simulink model "SMC_KI_s"  (R2023a)
settings: Solver=VariableStepAuto  StartTime=0.0  StopTime=10.0  RelTol=1e-3
undefined symbols (not defined in the file): C_col, DiscIntNeverNeededParam, J_col, K, k_I, k_sw, lambda, Phi, Tamax_table, Tamax_v_bp_ms, tau_f, Ts_ctrl
settings Model: Creator=Tan_Tram  LastModifiedBy=Tan_Tram

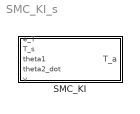
== system SMC_KI_s ==
  SMC_KI : Subsystem

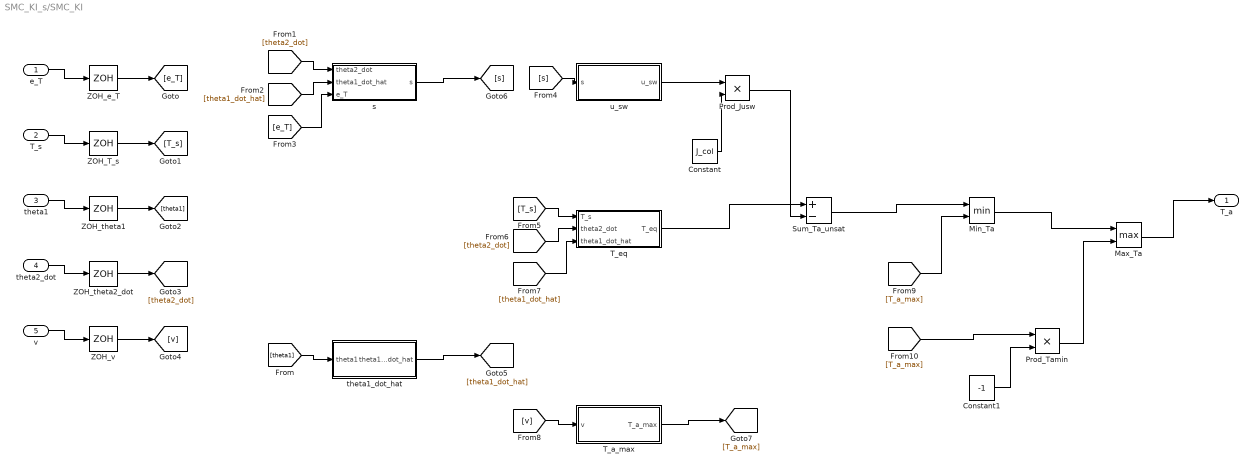
== system SMC_KI_s/SMC_KI ==
  e_T : Inport
  T_s : Inport  Port=2
  theta1 : Inport  Port=3
  theta2_dot : Inport  Port=4
  v : Inport  Port=5
  Constant : Constant  Value=J_col
  Constant1 : Constant  Value=-1
  Max_Ta : MinMax  Function=max  Inputs=2
  Min_Ta : MinMax  Inputs=2
  Prod_Jusw : Product  Inputs=**
  Prod_Tamin : Product  Inputs=**
  Sum_Ta_unsat : Sum  Inputs=+-
  T_a_max : Subsystem
  T_eq : Subsystem
  ZOH_T_s : ZeroOrderHold  SampleTime=Ts_ctrl
  ZOH_e_T : ZeroOrderHold  SampleTime=Ts_ctrl
  ZOH_theta1 : ZeroOrderHold  SampleTime=Ts_ctrl
  ZOH_theta2_dot : ZeroOrderHold  SampleTime=Ts_ctrl
  ZOH_v : ZeroOrderHold  SampleTime=Ts_ctrl
  s : Subsystem
  theta1_dot_hat : Subsystem
  u_sw : Subsystem
  T_a : Outport
  wires:
  e_T/1 -> ZOH_e_T/1
  ZOH_e_T/1 -> [e_T]
  T_s/1 -> ZOH_T_s/1
  ZOH_T_s/1 -> [T_s]
  theta1/1 -> ZOH_theta1/1
  ZOH_theta1/1 -> [theta1]
  theta2_dot/1 -> ZOH_theta2_dot/1
  ZOH_theta2_dot/1 -> [theta2_dot]
  v/1 -> ZOH_v/1
  ZOH_v/1 -> [v]
  [theta1] -> theta1_dot_hat/1(theta1)
  theta1_dot_hat/1(theta1_dot_hat) -> [theta1_dot_hat]
  [theta2_dot] -> s/1(theta2_dot)
  [theta1_dot_hat] -> s/2(theta1_dot_hat)
  [e_T] -> s/3(e_T)
  s/1(s) -> [s]
  [s] -> u_sw/1(s)
  [T_s] -> T_eq/1(T_s)
  [theta2_dot] -> T_eq/2(theta2_dot)
  [theta1_dot_hat] -> T_eq/3(theta1_dot_hat)
  u_sw/1(u_sw) -> Prod_Jusw/1
  Constant/1 -> Prod_Jusw/2
  T_eq/1(T_eq) -> Sum_Ta_unsat/1
  Prod_Jusw/1 -> Sum_Ta_unsat/2
  [v] -> T_a_max/1(v)
  T_a_max/1(T_a_max) -> [T_a_max]
  Sum_Ta_unsat/1 -> Min_Ta/1
  [T_a_max] -> Min_Ta/2
  [T_a_max] -> Prod_Tamin/1
  Constant1/1 -> Prod_Tamin/2
  Min_Ta/1 -> Max_Ta/1
  Prod_Tamin/1 -> Max_Ta/2
  Max_Ta/1 -> T_a/1

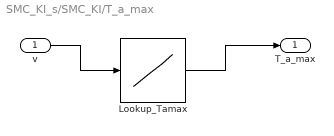
== system SMC_KI_s/SMC_KI/T_a_max ==
  v : Inport
  Lookup_Tamax : Lookup_n-D  NumberOfTableDimensions=1  BreakpointsForDimension1=Tamax_v_bp_ms  BreakpointsForDimension3=[5, 7]  Table=Tamax_table  ExtrapMethod=Clip  InternalRulePriority=Speed  RndMeth=Simplest
  T_a_max : Outport
  wires:
  v/1 -> Lookup_Tamax/1
  Lookup_Tamax/1 -> T_a_max/1

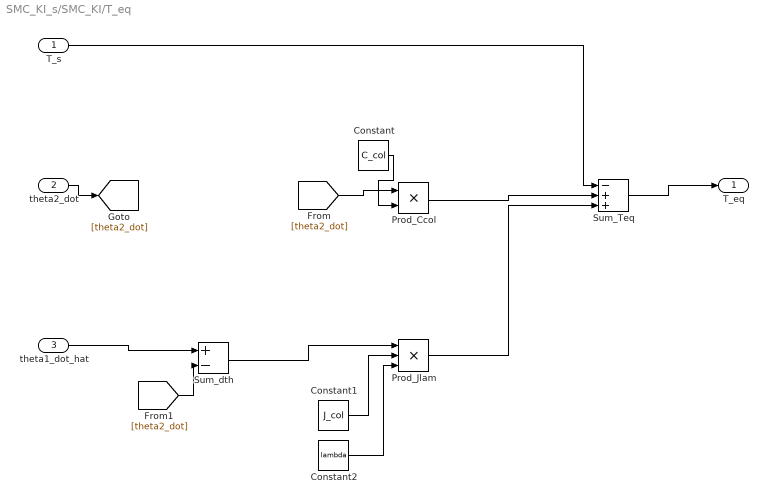
== system SMC_KI_s/SMC_KI/T_eq ==
  T_s : Inport
  theta2_dot : Inport  Port=2
  theta1_dot_hat : Inport  Port=3
  Constant : Constant  Value=C_col
  Constant1 : Constant  Value=J_col
  Constant2 : Constant  Value=lambda
  Prod_Ccol : Product  Inputs=**
  Prod_Jlam : Product  Inputs=***
  Sum_Teq : Sum  Inputs=-++
  Sum_dth : Sum  Inputs=+-
  T_eq : Outport
  wires:
  theta2_dot/1 -> [theta2_dot]
  [theta2_dot] -> Prod_Ccol/1
  Constant/1 -> Prod_Ccol/2
  theta1_dot_hat/1 -> Sum_dth/1
  [theta2_dot] -> Sum_dth/2
  Sum_dth/1 -> Prod_Jlam/1
  Constant1/1 -> Prod_Jlam/2
  Constant2/1 -> Prod_Jlam/3
  T_s/1 -> Sum_Teq/1
  Prod_Ccol/1 -> Sum_Teq/2
  Prod_Jlam/1 -> Sum_Teq/3
  Sum_Teq/1 -> T_eq/1

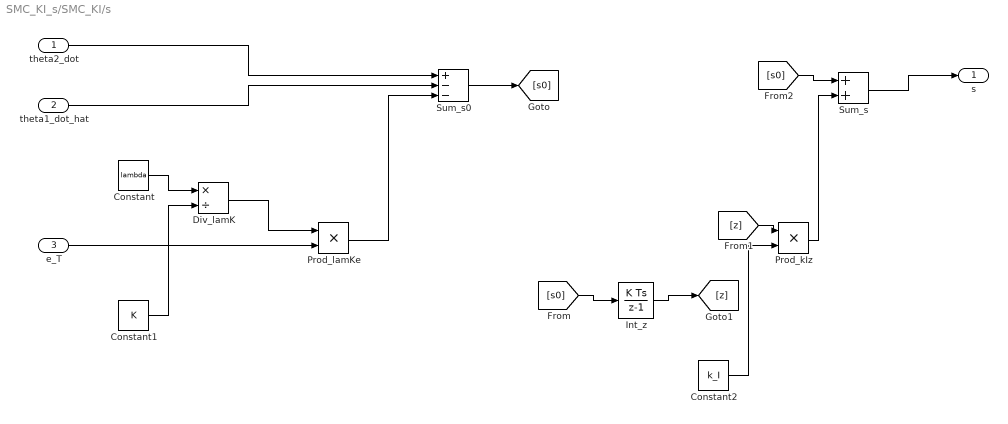
== system SMC_KI_s/SMC_KI/s ==
  theta2_dot : Inport
  theta1_dot_hat : Inport  Port=2
  e_T : Inport  Port=3
  Constant : Constant  Value=lambda
  Constant1 : Constant  Value=K
  Constant2 : Constant  Value=k_I
  Div_lamK : Product  Inputs=*/
  Int_z : DiscreteIntegrator  SampleTime=Ts_ctrl  LimitOutput=on  UpperSaturationLimit=Phi/k_I  LowerSaturationLimit=-Phi/k_I  ICPrevOutput=DiscIntNeverNeededParam  ICPrevScaledInput=DiscIntNeverNeededParam
  Prod_kIz : Product  Inputs=**
  Prod_lamKe : Product  Inputs=**
  Sum_s : Sum
  Sum_s0 : Sum  Inputs=+--
  s : Outport
  wires:
  Constant/1 -> Div_lamK/1
  Constant1/1 -> Div_lamK/2
  Div_lamK/1 -> Prod_lamKe/1
  e_T/1 -> Prod_lamKe/2
  theta2_dot/1 -> Sum_s0/1
  theta1_dot_hat/1 -> Sum_s0/2
  Prod_lamKe/1 -> Sum_s0/3
  Sum_s0/1 -> [s0]
  [s0] -> Int_z/1
  Int_z/1 -> [z]
  [z] -> Prod_kIz/1
  Constant2/1 -> Prod_kIz/2
  [s0] -> Sum_s/1
  Prod_kIz/1 -> Sum_s/2
  Sum_s/1 -> s/1

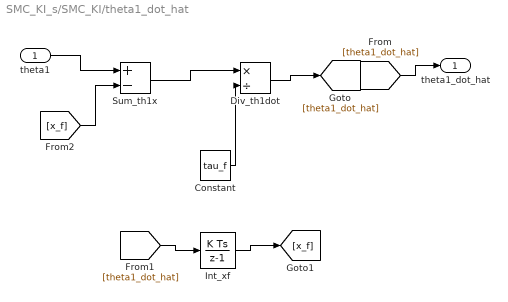
== system SMC_KI_s/SMC_KI/theta1_dot_hat ==
  theta1 : Inport
  Constant : Constant  Value=tau_f
  Div_th1dot : Product  Inputs=*/
  Int_xf : DiscreteIntegrator  SampleTime=Ts_ctrl  ICPrevOutput=DiscIntNeverNeededParam  ICPrevScaledInput=DiscIntNeverNeededParam
  Sum_th1x : Sum  Inputs=+-
  theta1_dot_hat : Outport
  wires:
  theta1/1 -> Sum_th1x/1
  [x_f] -> Sum_th1x/2
  Sum_th1x/1 -> Div_th1dot/1
  Constant/1 -> Div_th1dot/2
  Div_th1dot/1 -> [theta1_dot_hat]
  [theta1_dot_hat] -> theta1_dot_hat/1
  [theta1_dot_hat] -> Int_xf/1
  Int_xf/1 -> [x_f]

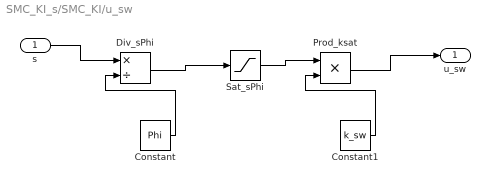
== system SMC_KI_s/SMC_KI/u_sw ==
  s : Inport
  Constant : Constant  Value=Phi
  Constant1 : Constant  Value=k_sw
  Div_sPhi : Product  Inputs=*/
  Prod_ksat : Product  Inputs=**
  Sat_sPhi : Saturate  UpperLimit=1  LowerLimit=-1
  u_sw : Outport
  wires:
  s/1 -> Div_sPhi/1
  Constant/1 -> Div_sPhi/2
  Div_sPhi/1 -> Sat_sPhi/1
  Sat_sPhi/1 -> Prod_ksat/1
  Constant1/1 -> Prod_ksat/2
  Prod_ksat/1 -> u_sw/1
